simulink model "chap4_1sim"  (Simulink 5.0)
settings: Solver=ode45  StartTime=0.0  StopTime=50  RelTol=1e-3
settings Model: LastModifiedBy=Administrator  ExtModeTrigMode=oneshot  ExtModeArmWhenConnect=off  LimitDataPoints=off  BooleanDataType=off

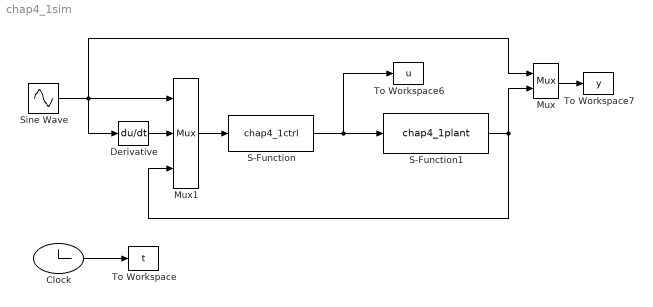
== system chap4_1sim ==
  Clock : Clock
  Derivative : Derivative
  Mux : Mux  Inputs=2
  Mux1 : Mux  Inputs=3
  S-Function : S-Function  FunctionName=chap4_1ctrl
  S-Function1 : S-Function  FunctionName=chap4_1plant
  Sine Wave : Sin  SampleTime=0
  To Workspace : ToWorkspace  VariableName=t  SampleTime=-1  SaveFormat=Array
  To Workspace6 : ToWorkspace  VariableName=u  SampleTime=-1  SaveFormat=Array
  To Workspace7 : ToWorkspace  VariableName=y  SampleTime=-1  SaveFormat=Array
  wires:
  Mux1/1 -> S-Function/1
  Mux/1 -> To Workspace7/1
  S-Function/1 -> S-Function1/1, To Workspace6/1
  Clock/1 -> To Workspace/1
  S-Function1/1 -> Mux/2, Mux1/3
  Derivative/1 -> Mux1/2
  Sine Wave/1 -> Mux/1, Mux1/1, Derivative/1
